simulink model "NEW_wbInterface"  (Simulink 7.9)
settings: Solver=FixedStepDiscrete  StartTime=0.0  StopTime=inf  FixedStep=1  RelTol=1e-3
settings Model: Creator=jorhabib  LastModifiedBy=jorhabib

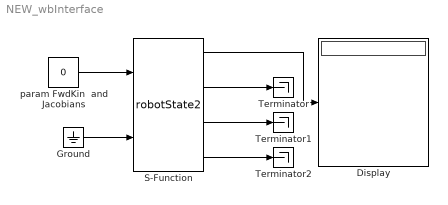
== system NEW_wbInterface ==
  Display : Display
  Ground : Ground
  S-Function : S-Function  FunctionName=robotState2  Parameters=val,robotname,localname  EnableBusSupport=off  mask{val=0, robotname='icubSim', localname='simulink'}
      mask prompts: robotname "rn"; localname "ln"
  Terminator : Terminator
  Terminator1 : Terminator
  Terminator2 : Terminator
  param FwdKin  and Jacobians : Constant  Value=0  OutDataTypeStr=int8  SampleTime=-1
  wires:
  param FwdKin  and Jacobians/1 -> S-Function/1
  Ground/1 -> S-Function/2
  S-Function/2 -> Terminator/1
  S-Function/3 -> Terminator1/1
  S-Function/4 -> Terminator2/1
  S-Function/1 -> Display/1
